simulink model "simulations"  (R2021b)
settings: Solver=VariableStepAuto  StartTime=0.0  StopTime=20  RelTol=1e-3
values from neighbouring files (symbols this model uses):
  A = zeros(n,n)    [comparacao.m]    (also in polinomial.m = Gz.den{1})
  B = zeros(n,1)    [comparacao.m]    (also in polinomial.m = Gz.num{1})
  C = num(2:end)    [comparacao.m]
  Gpid = (Kp + (tf([1 1], [1 -1], T)*Ki*T/2) + (tf([1 -1], [1 0], T)*Kd/T))    [sintese_direta.m]
  Gpol = tf(beta, alpha, T)    [polinomial.m]
  Gz = c2d(G, T, 'zoh')    [comparacao.m]    (also in espaco_estados.m; polinomial.m; sintese_direta.m)
  K = [0.110803158362 -0.502760127698 -0.0251684421391]    [K.mat]    (also in espaco_estados.m = fliplr(K(2:end)))
  n = n(2)-1    [comparacao.m]    (also in polinomial.m)
  P = -0.58728383282    [P.mat]    (also in polinomial.m = 1/dcgain(MF))
  T = 1    [comparacao.m]    (also in espaco_estados.m; polinomial.m; sintese_direta.m)
settings Model: Creator=Erick  LastModifiedBy=Erick

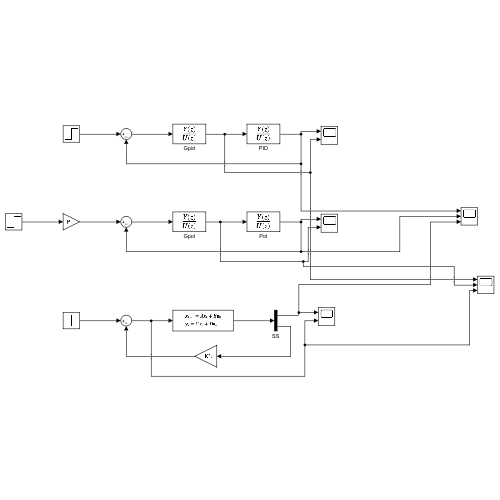
[thumbnail: Simulink's stored preview of the top-level diagram]
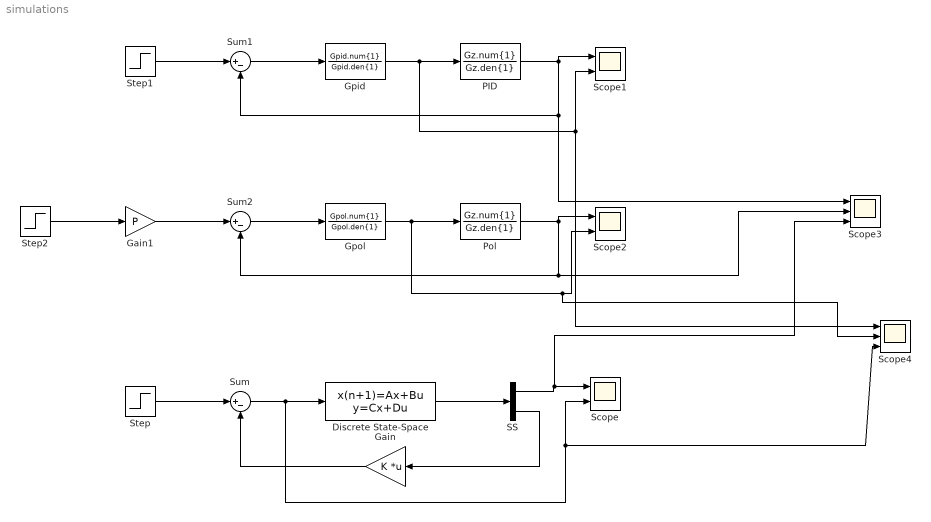
== system simulations ==
  Discrete State-Space : DiscreteStateSpace  A=A  B=B  C=[C;eye(n)]  D=zeros(n+1,1)  SampleTime=T
  Gain : Gain  Gain=K  Multiplication=Matrix(K*u)
  Gain1 : Gain  Gain=P
  Gpid : DiscreteTransferFcn  Numerator=Gpid.num{1}  Denominator=Gpid.den{1}
  Gpol : DiscreteTransferFcn  Numerator=Gpol.num{1}  Denominator=Gpol.den{1}
  PID : DiscreteTransferFcn  Numerator=Gz.num{1}  Denominator=Gz.den{1}
  Pol : DiscreteTransferFcn  Numerator=Gz.num{1}  Denominator=Gz.den{1}
  SS : Demux  Outputs=[1 3]
  Scope : Scope  NumInputPorts=2
  Scope1 : Scope  NumInputPorts=2
  Scope2 : Scope  NumInputPorts=2
  Scope3 : Scope  NumInputPorts=3
  Scope4 : Scope  NumInputPorts=3
  Step : Step  After=0.84  SampleTime=0
  Step1 : Step  SampleTime=0
  Step2 : Step  SampleTime=0
  Sum : Sum  Inputs=|+-
  Sum1 : Sum  Inputs=|+-
  Sum2 : Sum  Inputs=|+-
  wires:
  Discrete State-Space/1 -> SS/1
  SS/1 -> Scope3/3, Scope/1
  Sum/1 -> Scope/2, Scope4/3, Discrete State-Space/1
  SS/2 -> Gain/1
  Gain/1 -> Sum/2
  Step/1 -> Sum/1
  Gpid/1 -> Scope4/1, Scope1/2, PID/1
  Sum1/1 -> Gpid/1
  PID/1 -> Scope1/1, Scope3/1, Sum1/2
  Step1/1 -> Sum1/1
  Sum2/1 -> Gpol/1
  Gpol/1 -> Scope4/2, Scope2/2, Pol/1
  Pol/1 -> Scope2/1, Scope3/2, Sum2/2
  Gain1/1 -> Sum2/1
  Step2/1 -> Gain1/1
